simulink model "controller_nole"  (R2024b)
settings: Solver=VariableStepAuto  StartTime=0.0  StopTime=10.0  RelTol=1e-3
libraries: simulink x1, slpidlib x1, deeplib x1
settings Model: Creator=phama  LastModifiedBy=phama

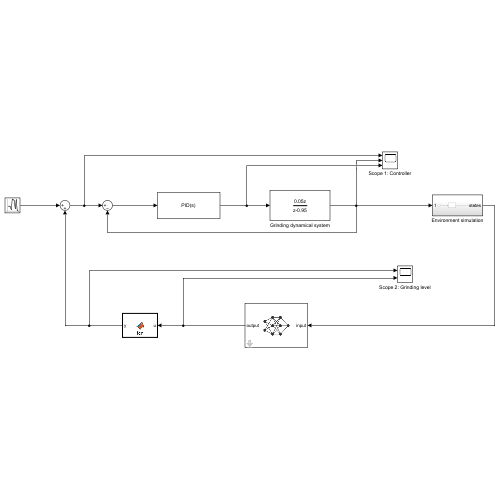
[thumbnail: Simulink's stored preview of the top-level diagram]
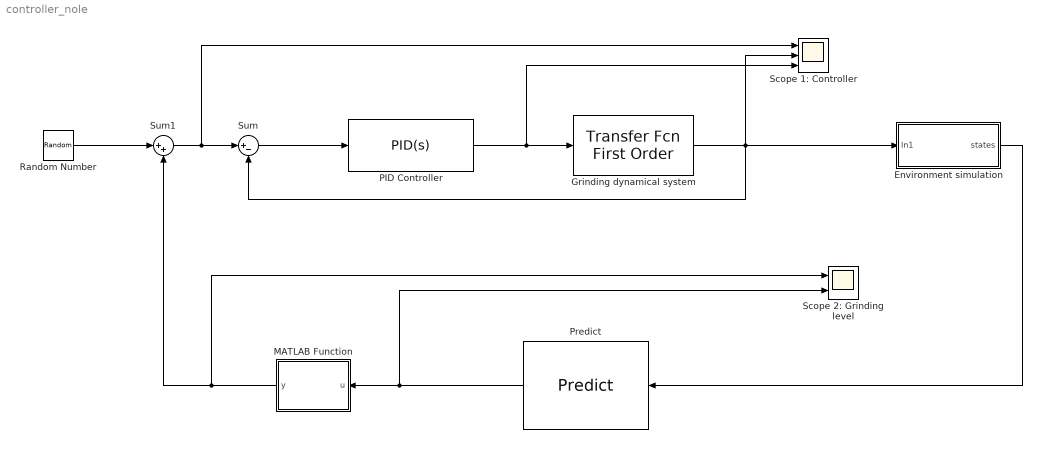
== system controller_nole ==
  Environment simulation : Subsystem
  Grinding dynamical system : simulink/Discrete/Transfer Fcn First Order  PoleZ=0.95  ICPrevOutput=0.0  DoSatur=off
  MATLAB Function : MATLAB Function  TreatAsAtomicUnit=on
  PID Controller : slpidlib/PID Controller  Controller=PID  Form=Parallel  TimeDomain=Continuous-time  UseExternalTs=off  SampleTime=-1  IntegratorMethod=Forward Euler  FilterMethod=Forward Euler  ControllerParametersSource=internal  P=1  I=1  UseKiTs=off  D=0  UseExternalDerivativeSource=off  N=100  UseFilter=on  TunerSelectOption=Transfer Function Based (PID Tuner App)  InitialConditionSource=internal  InitialConditionForIntegrator=0  InitialConditionForFilter=0  DifferentiatorICPrevScaledInput=0  ExternalReset=none  TrackingMode=off  Kt=1  LimitOutput=off  SatLimitsSource=internal  UpperSaturationLimit=inf  LowerSaturationLimit=-inf  LinearizeAsGain=on  AntiWindupMode=none  Kb=1  LimitIntegrator=off  UpperIntegratorSaturationLimit=inf  LowerIntegratorSaturationLimit=-inf  POutMin=[]  POutMax=[]  IOutMin=[]  IOutMax=[]  DOutMin=[]  DOutMax=[]  NOutMin=[]  NOutMax=[]  SumOutMin=[]  SumOutMax=[]  SaturationOutMin=[]  SaturationOutMax=[]  PParamMin=[]  PParamMax=[]  IParamMin=[]  IParamMax=[]  DParamMin=[]  DParamMax=[]  NParamMin=[]  NParamMax=[]  KbParamMin=[]  KbParamMax=[]  KtParamMin=[]  KtParamMax=[]  KbOutMin=[]  KbOutMax=[]  KtOutMin=[]  KtOutMax=[]  IntegratorOutMin=[]  IntegratorOutMax=[]  FilterOutMin=[]  FilterOutMax=[]  SumI1OutMin=[]  SumI1OutMax=[]  SumI2OutMin=[]  SumI2OutMax=[]  SumI3OutMin=[]  SumI3OutMax=[]  SumI4OutMin=[]  SumI4OutMax=[]  SumDOutMin=[]  SumDOutMax=[]  DifferentiatorOutMin=[]  DifferentiatorOutMax=[]  FilterDiffOutCoefMin=[]  FilterDiffOutCoefMax=[]  ReciprocalOutMin=[]  ReciprocalOutMax=[]  SumDenOutMin=[]  SumDenOutMax=[]  SumNumOutMin=[]  SumNumOutMax=[]  DivideOutMin=[]  DivideOutMax=[]  UdiffTsProdOutMin=[]  UdiffTsProdOutMax=[]  NTsProdOutMin=[]  NTsProdOutMax=[]  UintegralTsProdOutMin=[]  UintegralTsProdOutMax=[]  UngainTsProdOutMin=[]  UngainTsProdOutMax=[]  ClampingZeroOutDataTypeStr=Inherit: Inherit via back propagation  ClampingZeroOutMin=[]  ClampingZeroOutMax=[]  FilterDenConstantOutDataTypeStr=Inherit: Inherit via back propagation  FilterDenConstantOutMin=[]  FilterDenConstantOutMax=[]  PCopyOutDataTypeStr=Inherit: Inherit via back propagation  PCopyOutMin=[]  PCopyOutMax=[]  NCopyOutDataTypeStr=Inherit: Inherit via back propagation  NCopyOutMin=[]  NCopyOutMax=[]  IntegratorContinuousStateAttributes=''  IntegratorStateMustResolveToSignalObject=off  IntegratorRTWStateStorageClass=Auto  FilterContinuousStateAttributes=''  FilterStateMustResolveToSignalObject=off  FilterRTWStateStorageClass=Auto  ParallelPVariant=InternalParameters  IdealPVariant=Disabled  IVariant=InternalParameters  DVariant=InternalParameters  IntegratorVariant=Continuous  SatVariant=Disabled  AWVariant=Passthrough  PCopyVariant=Disabled  TRVariant=Disabled  FdbkBlocksVariant=Forward  IdealPFdbkVariant=Disabled  SatFdbkVariant=Disabled  DerivativeFilterVariant=ContFilter  NVariant=InternalParameters  NCopyVariant=Disabled  FilterICVariant=InternalICsFilter  IntegratorICVariant=InternalICs  ExternalResetVariant=Disabled  TRSumVariant=Passthrough  SumFdbkVariant=Disabled  SumVariant=Sum_PID  TsampFilterVariant=InternalTs  TsampNgainVariant=Passthrough  TsampIntegralVariant=Disabled_SignalSpec  ExternalSaturationOutDataTypeStr=Inherit: Same as second input  DerivativeSourceVariant=ErrorSignal  PreIntVariant=InternalPreInt
  Predict : deeplib/Predict  Network=Network from MAT-file  NetworkFunction=squeezenet  NetworkFilePath=untitled.mat  MiniBatchSize=128  InputDataFormats={'',''}  Predictions=on  Activations={}  ForceInterpretedSim=off  EnableDLNetwork=on  LastKnownNetworkFilePath=''  LastKnownNetworkTimeStamp=''
  Random Number : RandomNumber  SampleTime=0.1
  Scope 1: Controller : Scope  NumInputPorts=3
  Scope 2: Grinding level : Scope  NumInputPorts=2
  Sum : Sum  Inputs=|+-
  Sum1 : Sum  Inputs=|++
  wires:
  PID Controller/1 -> Scope 1: Controller/3, Grinding dynamical system/1
  Sum/1 -> PID Controller/1
  Grinding dynamical system/1 -> Sum/2, Environment simulation/1(In1), Scope 1: Controller/2
  Sum1/1 -> Scope 1: Controller/1, Sum/1
  Random Number/1 -> Sum1/1
  MATLAB Function/1(y) -> Scope 2: Grinding level/1, Sum1/2
  Environment simulation/1(states) -> Predict/1
  Predict/1 -> Scope 2: Grinding level/2, MATLAB Function/1(u)

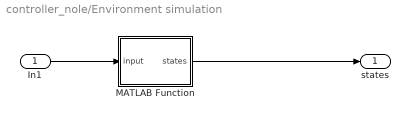
== system controller_nole/Environment simulation ==
  In1 : Inport
  MATLAB Function : MATLAB Function  TreatAsAtomicUnit=on
  states : Outport
  wires:
  In1/1 -> MATLAB Function/1(input)
  MATLAB Function/1(states) -> states/1

== matlab function controller_nole/Environment simulation/MATLAB Function ==
  data: input input; states output
function states = environment(input)
    %#codegen

    % Define how each state is computed from the input
    states = zeros(6, 1); % Pre-allocate the output array
    states(1) = input * 2;            % State 1
    states(2) = input ^ 2;            % State 2
    states(3) = sin(input);           % State 3
    states(4) = cos(input);           % State 4
    states(5) = log(1 + abs(input));  % State 5
    states(6) = exp(-input);          % State 6
end

== matlab function controller_nole/MATLAB Function ==
  data: u input; y output
function y = fcn(u)
%#codegen

% Specify the base value and delta
base_value = 0;   % Starting intensity
delta = 10;       % Step size for each level

% Check the input and assign the output based on 20 cases
if u == 1
    y = base_value;
elseif u == 2
    y = base_value + 1 * delta;
elseif u == 3
    y = base_value + 2 * delta;
elseif u == 4
    y = base_value + 3 * delta;
elseif u == 5
    y = base_value + 4 * delta;
elseif u == 6
    y = base_value + 5 * delta;
elseif u == 7
    y = base_value + 6 * delta;
elseif u == 8
    y = base_value + 7 * delta;
elseif u == 9
    y = base_value + 8 * delta;
elseif u == 10
    y = base_value + 9 * delta;
elseif u == 11
    y = base_value + 10 * delta;
elseif u == 12
    y = base_value + 11 * delta;
elseif u == 13
    y = base_value + 12 * delta;
elseif u == 14
    y = base_value + 13 * delta;
elseif u == 15
    y = base_value + 14 * delta;
elseif u == 16
    y = base_value + 15 * delta;
elseif u == 17
    y = base_value + 16 * delta;
elseif u == 18
    y = base_value + 17 * delta;
elseif u == 19
    y = base_value + 18 * delta;
elseif u == 20
    y = base_value + 19 * delta;
else
    y = 0; % Default value for out-of-range inputs
end
